simulink library "HndPosSts"  (R2022a)
settings: Solver=VariableStepAuto  StartTime=0.0  StopTime=10.0  RelTol=1e-3
settings Model: Creator=DELL  LastModifiedBy=DELL

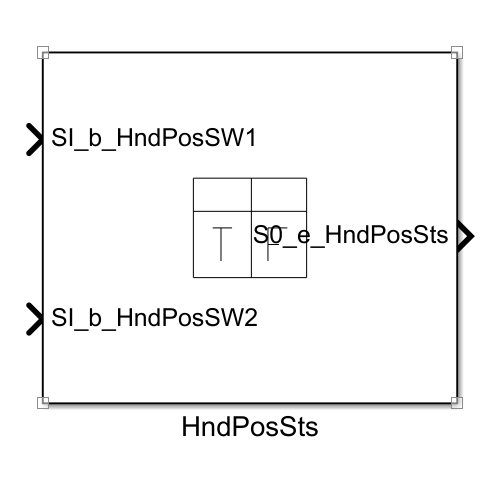
[thumbnail: Simulink's stored preview of the top-level diagram]
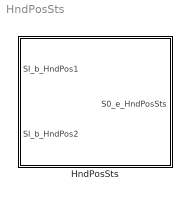
== system HndPosSts ==
  HndPosSts : Truth Table  TreatAsAtomicUnit=on

== matlab function HndPosSts/HndPosSts ==
  data: SI_b_HndPos1 input boolean; S0_e_HndPosSts output uint8; SI_b_HndPos2 input boolean
function S0_e_HndPosSts = fcn(SI_b_HndPos1, SI_b_HndPos2)

aVarTruthTableCondition_1 = false;
aVarTruthTableCondition_2 = false;


% condition 1

aVarTruthTableCondition_1 = logical(SI_b_HndPos1 == 1);

% condition 2

aVarTruthTableCondition_2 = logical(SI_b_HndPos2 == 1);

if (~aVarTruthTableCondition_1 && ~aVarTruthTableCondition_2)
    aFcnTruthTableAction_1();
elseif (aVarTruthTableCondition_1 && aVarTruthTableCondition_2)
    aFcnTruthTableAction_2();
elseif (aVarTruthTableCondition_1 && ~aVarTruthTableCondition_2)
    aFcnTruthTableAction_3();
else % Default
    aFcnTruthTableAction_4();
end

function aFcnTruthTableAction_1()

% All Fold

SO_e_HndPosSts = 0;

function aFcnTruthTableAction_2()

% ALL Unfold

SO_e_HndPosSts = 1;

function aFcnTruthTableAction_3()

% Half Unfold

SO_e_HndPosSts = 2;

function aFcnTruthTableAction_4()

% Error

SO_e_HndPosSts = 3;
